simulink model "HDLHeaderFull"  (R2024a)
settings: Solver=FixedStepDiscrete  StartTime=0.0  StopTime=stopTime  RelTol=1e-3
undefined symbols (not defined in the file or in its folder): CONST, paramFile
libraries: dspsrcs4 x5, HDL_ieee_8021513 x2, hdlsllib x1, whdlutilities x1
settings Model: DataTypeOverride=Off  Creator=cotti  LastModifiedBy=cotti
settings OptimizationCC: BlockReduction=off  ConditionallyExecuteInputs=off  DefaultParameterBehavior=Inlined  InheritOutputTypeSmallerThanSingle=on
settings DebuggingCC: AlgebraicLoopMsg=error  ArtificialAlgebraicLoopMsg=error  SingleTaskRateTransMsg=error  UnconnectedInputMsg=warning  UnconnectedOutputMsg=warning  UnconnectedLineMsg=warning
settings HardwareCC: ProdBitPerPointer=32  ProdBitPerSizeT=32  ProdBitPerPtrDiffT=32  ProdLargestAtomicFloat=None  ProdIntDivRoundTo=Undefined  ProdEndianess=Unspecified  ProdWordSize=32  ProdHWDeviceType=ASIC/FPGA->ASIC/FPGA  TargetBitPerLong=64  TargetBitPerPointer=64  TargetBitPerSizeT=64  TargetBitPerPtrDiffT=64  TargetLongLongMode=on  TargetIntDivRoundTo=Zero  TargetEndianess=LittleEndian  TargetWordSize=64  TargetHWDeviceType=Custom Processor->MATLAB Host Computer  ProdEqTarget=off

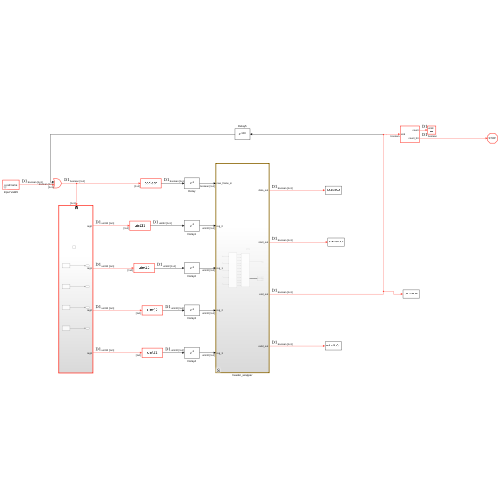
[thumbnail: Simulink's stored preview of the top-level diagram]
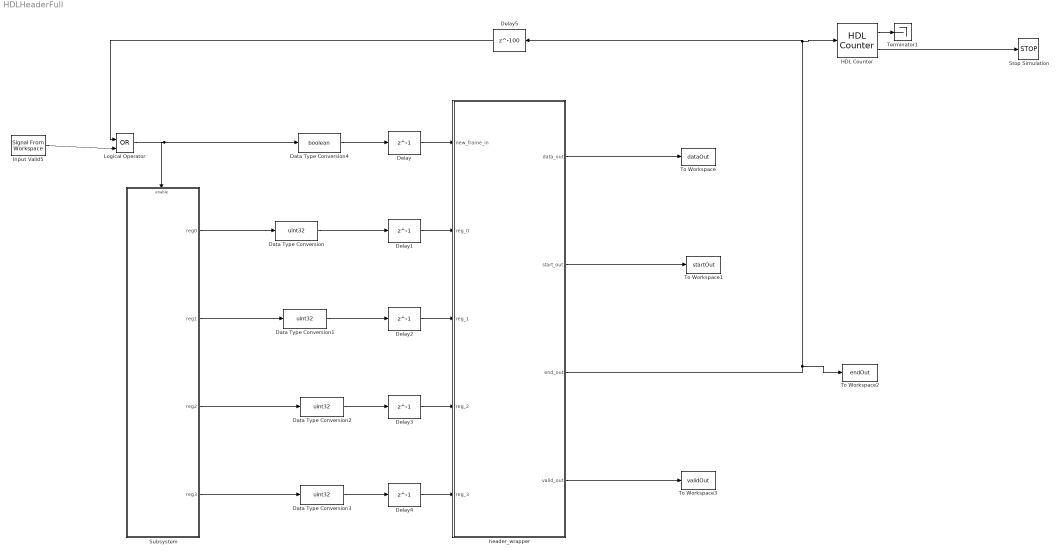
== system HDLHeaderFull ==
  Data Type Conversion{,1..3} (4 alike) : DataTypeConversion  OutDataTypeStr=uint32  SaturateOnIntegerOverflow=off  RndMeth=Floor
  Data Type Conversion4 : DataTypeConversion  OutDataTypeStr=boolean  SaturateOnIntegerOverflow=off  RndMeth=Floor
  Delay{,1..4} (5 alike) : Delay  DelayLength=1  InitialCondition=0  UseCircularBuffer=on
  Delay5 : Delay  DelayLength=100  InitialCondition=0  UseCircularBuffer=on
  HDL Counter : hdlsllib/Sources/HDL Counter  CountType=Count limited  CountInit=0  CountStep=1  CountMax=length(paramFile)  CountFromType=Initial value  CountFrom=0  CountResetPort=off  CountLoadPort=off  CountEnbPort=on  CountDirPort=off  CountHitOutputPort=on  CountDataType=Unsigned  CountWordLen=8  CountFracLen=0  CountSampTime=1
  Input Valid5 : dspsrcs4/Signal From Workspace  X=newFrame  Ts=1/CONST.fDAC  nsamps=1  OutputAfterFinalValue=Setting to zero  ignoreOrWarnInputAndFrameLengths=off  OutputFrames=off
  Logical Operator : Logic  Operator=OR  IconShape=distinctive  AllPortsSameDT=off  OutDataTypeStr=boolean
  Stop Simulation : Stop
  Subsystem : Subsystem
  Terminator1 : Terminator
  To Workspace : ToWorkspace  VariableName=dataOut  SampleTime=1/CONST.fs
      settings: Save2DSignal=2-D array (concatenate along first dimension)
  To Workspace1 : ToWorkspace  VariableName=startOut  SampleTime=1/CONST.fs
      settings: Save2DSignal=2-D array (concatenate along first dimension)
  To Workspace2 : ToWorkspace  VariableName=endOut  SampleTime=1/CONST.fs
      settings: Save2DSignal=2-D array (concatenate along first dimension)
  To Workspace3 : ToWorkspace  VariableName=validOut  SampleTime=1/CONST.fs
      settings: Save2DSignal=2-D array (concatenate along first dimension)
  header_wrapper : Subsystem  TreatAsAtomicUnit=on
  wires:
  Data Type Conversion/1 -> Delay1/1
  Data Type Conversion1/1 -> Delay2/1
  Data Type Conversion2/1 -> Delay3/1
  Data Type Conversion3/1 -> Delay4/1
  Data Type Conversion4/1 -> Delay/1
  Logical Operator/1 -> Subsystem/Enable, Data Type Conversion4/1
  Input Valid5/1 -> Logical Operator/2
  header_wrapper/3(end_out) -> Delay5/1, HDL Counter/1, To Workspace2/1
  Subsystem/1(reg0) -> Data Type Conversion/1
  Subsystem/2(reg1) -> Data Type Conversion1/1
  Subsystem/3(reg2) -> Data Type Conversion2/1
  Subsystem/4(reg3) -> Data Type Conversion3/1
  HDL Counter/1 -> Terminator1/1
  HDL Counter/2 -> Stop Simulation/1
  header_wrapper/1(data_out) -> To Workspace/1
  header_wrapper/2(start_out) -> To Workspace1/1
  header_wrapper/4(valid_out) -> To Workspace3/1
  Delay/1 -> header_wrapper/1(new_frame_in)
  Delay1/1 -> header_wrapper/2(reg_0)
  Delay2/1 -> header_wrapper/3(reg_1)
  Delay3/1 -> header_wrapper/4(reg_2)
  Delay4/1 -> header_wrapper/5(reg_3)
  Delay5/1 -> Logical Operator/1

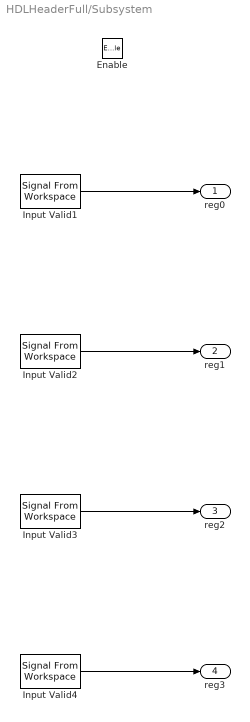
== system HDLHeaderFull/Subsystem ==
  Enable : EnablePort
  Input Valid1 : dspsrcs4/Signal From Workspace  X=reg0  Ts=1/CONST.fDAC  nsamps=1  OutputAfterFinalValue=Setting to zero  ignoreOrWarnInputAndFrameLengths=off  OutputFrames=off
  Input Valid2 : dspsrcs4/Signal From Workspace  X=reg1  Ts=1/CONST.fDAC  nsamps=1  OutputAfterFinalValue=Setting to zero  ignoreOrWarnInputAndFrameLengths=off  OutputFrames=off
  Input Valid3 : dspsrcs4/Signal From Workspace  X=reg2  Ts=1/CONST.fDAC  nsamps=1  OutputAfterFinalValue=Setting to zero  ignoreOrWarnInputAndFrameLengths=off  OutputFrames=off
  Input Valid4 : dspsrcs4/Signal From Workspace  X=reg3  Ts=1/CONST.fDAC  nsamps=1  OutputAfterFinalValue=Setting to zero  ignoreOrWarnInputAndFrameLengths=off  OutputFrames=off
  reg0 : Outport
  reg1 : Outport  Port=2
  reg2 : Outport  Port=3
  reg3 : Outport  Port=4
  wires:
  Input Valid3/1 -> reg2/1
  Input Valid2/1 -> reg1/1
  Input Valid4/1 -> reg3/1
  Input Valid1/1 -> reg0/1

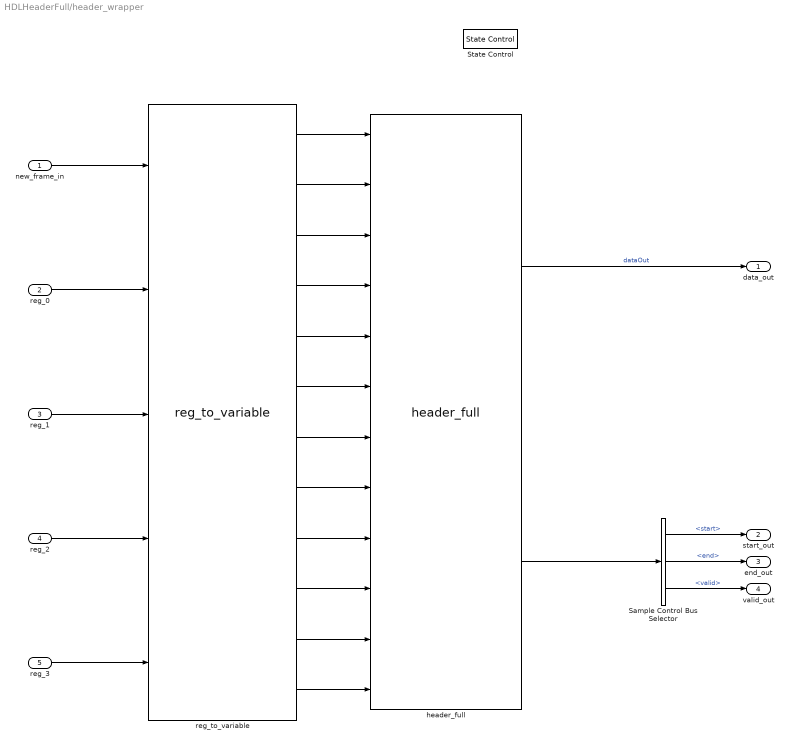
== system HDLHeaderFull/header_wrapper ==
  new_frame_in : Inport
  reg_0 : Inport  Port=2
  reg_1 : Inport  Port=3
  reg_2 : Inport  Port=4
  reg_3 : Inport  Port=5
  Sample Control Bus Selector : whdlutilities/Sample Control Bus Selector  OutputSignals=start,end,valid
  State Control : StateControl  StateControl=Synchronous
  header_full : HDL_ieee_8021513/header_full  SystemSampleTime=-1  VariantActivationTime=update diagram  AllowFlexibleInterface=on  Latency=0  AutoFrameSizeCalculation=off
      settings: LibrarySourceBlock=|
      | hdlsllib/Ports &
      | Subsystems/Subsystem
  reg_to_variable : HDL_ieee_8021513/reg_to_variable  SystemSampleTime=-1  VariantActivationTime=update diagram  AllowFlexibleInterface=on  Latency=0  AutoFrameSizeCalculation=off
      settings: SourceProductName=HDL IEEE 8021513
  data_out : Outport
  start_out : Outport  Port=2  VectorParamsAs1DForOutWhenUnconnected=off
  end_out : Outport  Port=3  VectorParamsAs1DForOutWhenUnconnected=off
  valid_out : Outport  Port=4  VectorParamsAs1DForOutWhenUnconnected=off
  wires:
  header_full/1 -> data_out/1  "dataOut"
  header_full/2 -> Sample Control Bus Selector/1
  Sample Control Bus Selector/1 -> start_out/1  "<start>"
  Sample Control Bus Selector/2 -> end_out/1  "<end>"
  Sample Control Bus Selector/3 -> valid_out/1  "<valid>"
  reg_to_variable/12 -> header_full/12
  reg_to_variable/11 -> header_full/11
  reg_to_variable/10 -> header_full/10
  reg_to_variable/9 -> header_full/9
  reg_to_variable/8 -> header_full/8
  reg_to_variable/7 -> header_full/7
  reg_to_variable/6 -> header_full/6
  reg_to_variable/5 -> header_full/5
  reg_to_variable/4 -> header_full/4
  reg_to_variable/3 -> header_full/3
  reg_to_variable/2 -> header_full/2
  reg_to_variable/1 -> header_full/1
  new_frame_in/1 -> reg_to_variable/1
  reg_0/1 -> reg_to_variable/2
  reg_1/1 -> reg_to_variable/3
  reg_2/1 -> reg_to_variable/4
  reg_3/1 -> reg_to_variable/5
